simulink model "pidmanuel"  (R2024a)
settings: Solver=VariableStepAuto  StartTime=0.0  StopTime=800  RelTol=1e-3
settings Model: Creator=sabri  LastModifiedBy=sabri

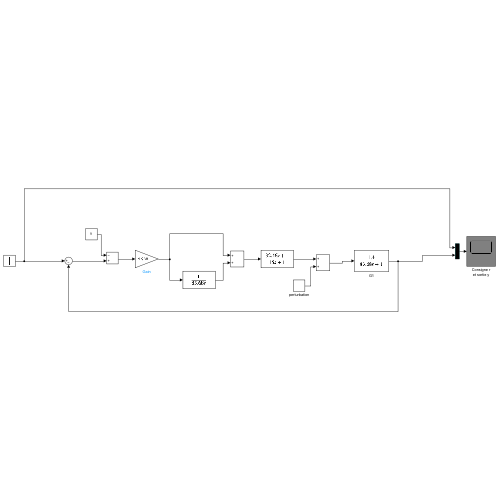
[thumbnail: Simulink's stored preview of the top-level diagram]
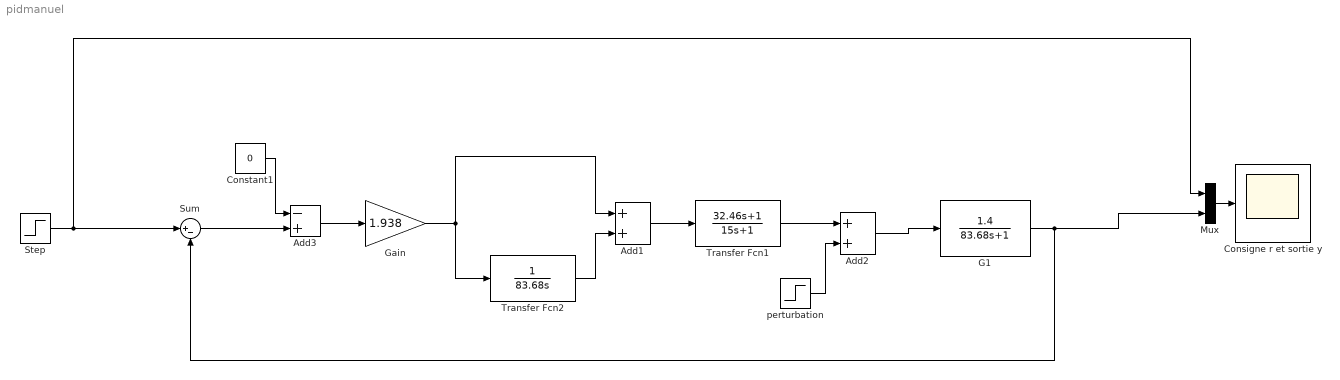
== system pidmanuel ==
  Add1 : Sum
  Add2 : Sum
  Add3 : Sum  Inputs=-+
  Consigne r et sortie y : Scope
  Constant1 : Constant  Value=0
  G1 : TransferFcn  Numerator=[1.4]  Denominator=[83.68 1]
  Gain : Gain  Gain=1.938
  Mux : Mux  Inputs=2
  Step : Step  Time=10  After=7.8  SampleTime=0
  Sum : Sum  Inputs=|+-
  Transfer Fcn1 : TransferFcn  Numerator=[32.46 1]  Denominator=[15 1]
  Transfer Fcn2 : TransferFcn  Denominator=[83.68 0]
  perturbation : Step  Time=10  After=15  SampleTime=0
  wires:
  Step/1 -> Mux/1, Sum/1
  Mux/1 -> Consigne r et sortie y/1
  Add3/1 -> Gain/1
  Sum/1 -> Add3/2
  Constant1/1 -> Add3/1
  Gain/1 -> Transfer Fcn2/1, Add1/1
  Transfer Fcn2/1 -> Add1/2
  Add1/1 -> Transfer Fcn1/1
  G1/1 -> Mux/2, Sum/2
  Transfer Fcn1/1 -> Add2/1
  Add2/1 -> G1/1
  perturbation/1 -> Add2/2
